simulink model "RobotX_August20"  (R2014a)
settings: Solver=FixedStepDiscrete  StartTime=0.0  StopTime=inf  FixedStep=.1  RelTol=1e-3
undefined symbols (not defined in the file): Com1, Com2, Com3, Com4, DiscIntNeverNeededParam
libraries: xpcseriallib x8, simulink x4, speedgoatlib_IO102 x1, slrtlib x1
(part 2 of 2)

== matlab function RobotX_August20/Main FSM/Main Task Option/Message Composer ==
  data: taskStrInit input; taskStrAdj output
function taskStrAdj = composeMessage(taskStrInit)
%Written by Anderson Lebbad on August 9, 2013
%Last Edited: Edward Zhu on June 2, 2014

%This function adjusts the length of a vector to a set value by filling
%the remaining space with 0's. This is necessary for data store objects
%that have a fixed size for the memory allocation, but a variable length
%input.

%Length of message packet
strLength = 8;

%Size of text in message
taskStrLength = size(taskStrInit,1);

%Pad end of text with zeros
taskStrAdj = [taskStrInit' zeros(1,strLength-taskStrLength)];

== matlab function RobotX_August20/Parameters/GPS Points/GPS Selector ==
  data: course input; ssGate output; rtnIn input; ssGateA input; transWptA input; obstNavStartA input; obstNavEndA input; acouLocA input; dockA input; ssGateB input; transWptB input; obstNavStartB input; obstNavEndB input; acouLocB input; dockB input; ssGateT input; transWptT input; obstNavStartT input; obstNavEndT input; acouLocT input; dockT input; transWpt output; obstNavStart output; obstNavEnd output; acouLoc output; dock output; rtnOut output
function [ssGate,transWpt,obstNavStart,obstNavEnd,acouLoc,dock,rtnOut] = ...
    GPSselector(course,rtnIn,...
    ssGateA,transWptA,obstNavStartA,obstNavEndA,acouLocA,dockA,...
    ssGateB,transWptB,obstNavStartB,obstNavEndB,acouLocB,dockB,...
    ssGateT,transWptT,obstNavStartT,obstNavEndT,acouLocT,dockT)

%Written by: Anderson Lebbad on July 18, 2013
%Last Edited: Edward Zhu on June
%   Data type mismatch addressed
%   Character conversion redundant

%Selects GPS Points to use based on input Course

%Check value of CourseStr and pass inputs accordingly

switch course
    case uint8('A')
        ssGate = ssGateA;
        transWpt = transWptA;
        obstNavStart = obstNavStartA;
        obstNavEnd = obstNavEndA;
        acouLoc = acouLocA;
        dock = dockA;
        rtnOut = rtnIn;
        
    case uint8('B')
        ssGate = ssGateB;
        transWpt = transWptB;
        obstNavStart = obstNavStartB;
        obstNavEnd = obstNavEndB;
        acouLoc = acouLocB;
        dock = dockB;
        rtnOut = rtnIn;
        
    otherwise
        ssGate = ssGateT;
        transWpt = transWptT;
        obstNavStart = obstNavStartT;
        obstNavEnd = obstNavEndT;
        acouLoc = acouLocT;
        dock = dockT;
        rtnOut = rtnIn;
end
